simulink model "Hoist_raw"  (R2015b)
settings: Solver=ode23t  StartTime=0.0  StopTime=10  MaxStep=0.2  RelTol=1e-3
undefined symbols (not defined in the file or in its folder): sigbuilder_block
libraries: fl_lib x16, nesl_utility x4
settings Model: Creator=OlgeirMac  LastModifiedBy=OlgeirMac
settings SolverCC: ZeroCrossControl=EnableAll

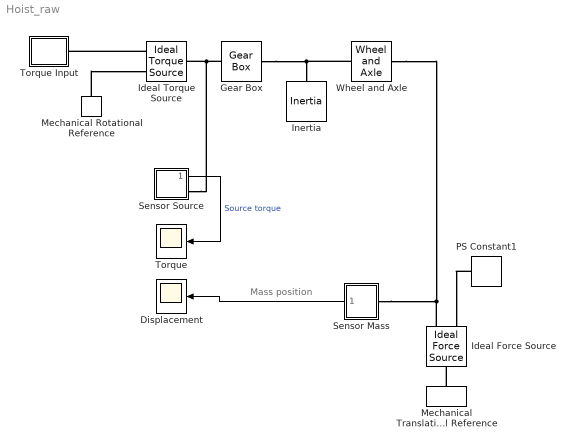
== system Hoist_raw ==
  note: Mass position
  Displacement : Scope
  Gear Box : fl_lib/Mechanical/Mechanisms/Gear Box  ratio=5  t_in_specify=off  t_in_priority=None  t_in=0 N*m  t_out_specify=off  t_out_priority=None  t_out=0 N*m
  Ideal Force Source : fl_lib/Mechanical/Mechanical Sources/Ideal Force Source
  Ideal Torque Source : fl_lib/Mechanical/Mechanical Sources/Ideal Torque Source
  Inertia : fl_lib/Mechanical/Rotational Elements/Inertia  inertia=0.001 kg*m^2  w_specify=off  w_priority=None  w=0 rad/s  t_specify=off  t_priority=None  t=0 N*m
  Mechanical Rotational Reference : fl_lib/Mechanical/Rotational Elements/Mechanical Rotational Reference
  Mechanical Translational Reference : fl_lib/Mechanical/Translational Elements/Mechanical Translational Reference
  PS Constant1 : fl_lib/Physical Signals/Sources/PS Constant  constant=9.8*load
  Sensor Mass : Subsystem
      mask Display: disp('P')
  Sensor Source : Subsystem
      mask Display: disp('P')
  Torque : Scope
  Torque Input : Subsystem
  Wheel and Axle : fl_lib/Mechanical/Mechanisms/Wheel and Axle  R=0.5 m  or=1  orient=1  t_specify=off  t_priority=None  t=0 N*m  f_specify=off  f_priority=None  f=0 N
  wires:
  Sensor Mass/1(Out1) -> Displacement/1
  Sensor Source/1(Out1) -> Torque/1  "Source torque"
  connections:
  Ideal Torque Source/RConn1 -- Torque Input/RConn1
  Gear Box/LConn1 -- Sensor Source/RConn1 -- Ideal Torque Source/LConn1
  Gear Box/RConn1 -- Wheel and Axle/LConn1 -- Inertia/LConn1
  Mechanical Rotational Reference/LConn1 -- Ideal Torque Source/RConn2
  Sensor Mass/LConn1 -- Wheel and Axle/RConn1 -- Ideal Force Source/RConn2
  PS Constant1/RConn1 -- Ideal Force Source/RConn1
  Mechanical Translational Reference/LConn1 -- Ideal Force Source/LConn1

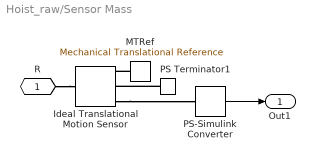
== system Hoist_raw/Sensor Mass ==
  Ideal Translational Motion Sensor : fl_lib/Mechanical/Mechanical Sensors/Ideal Translational Motion Sensor  Tag=Factory Generic  offset=0 m
  MTRef : fl_lib/Mechanical/Translational Elements/Mechanical Translational Reference  Tag=Factory Generic
  PS Terminator1 : fl_lib/Physical Signals/Sinks/PS Terminator
  PS-Simulink Converter : nesl_utility/PS-Simulink Converter  PhysicalDomain=network_engine_domain  SubClassName=ps_output  LeftPortType=input  RightPortType=output  PseudoPeriodic=off  Frequencies=[]  Unit=1  AffineConversion=off
  R : PMIOPort  Port=1  Side=Left
  Out1 : Outport
  wires:
  PS-Simulink Converter/1 -> Out1/1
  connections:
  Ideal Translational Motion Sensor/RConn3 -- PS-Simulink Converter/LConn1
  MTRef/LConn1 -- Ideal Translational Motion Sensor/RConn1
  R/RConn1 -- Ideal Translational Motion Sensor/LConn1
  PS Terminator1/LConn1 -- Ideal Translational Motion Sensor/RConn2

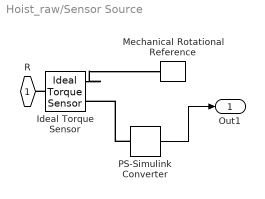
== system Hoist_raw/Sensor Source ==
  Ideal Torque Sensor : fl_lib/Mechanical/Mechanical Sensors/Ideal Torque Sensor
  Mechanical Rotational Reference : fl_lib/Mechanical/Rotational Elements/Mechanical Rotational Reference
  PS-Simulink Converter : nesl_utility/PS-Simulink Converter  PhysicalDomain=network_engine_domain  SubClassName=ps_output  LeftPortType=input  RightPortType=output  PseudoPeriodic=off  Frequencies=[]  Unit=1  AffineConversion=off
  R : PMIOPort  Port=1  Side=Right
  Out1 : Outport
  wires:
  PS-Simulink Converter/1 -> Out1/1
  connections:
  Ideal Torque Sensor/LConn1 -- R/RConn1
  Ideal Torque Sensor/RConn1 -- Mechanical Rotational Reference/LConn1
  PS-Simulink Converter/LConn1 -- Ideal Torque Sensor/RConn2

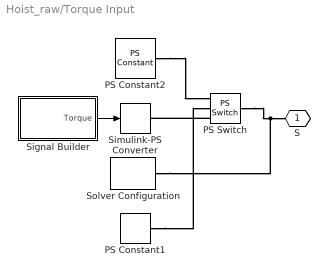
== system Hoist_raw/Torque Input ==
  PS Constant1 : fl_lib/Physical Signals/Sources/PS Constant  constant=2
  PS Constant2 : fl_lib/Physical Signals/Sources/PS Constant  constant=0
  PS Switch : fl_lib/Physical Signals/Nonlinear Operators/PS Switch  Threshold=1
  Signal Builder : Subsystem  Tag=STV Subsys  LoadFcn=sigbuilder_block('load');  StartFcn=sigbuilder_block('start');  StopFcn=sigbuilder_block('stop');  ClipboardFcn=sigbuilder_block('clipboard');  mask(Sigbuilder block){}
      mask help: Sigbuilder GUI
      mask init:
      | if ~strcmp(get_param(bdroot(gcbh),'SimulationStatus'),'stopped') tuvar = sigbuilder_block('maskInit'); end
      settings: CopyFcn=sigbuilder_block('copy');  DeleteFcn=sigbuilder_block('delete');  ModelCloseFcn=sigbuilder_block('modelClose');  PreSaveFcn=sigbuilder_block('preSave');  PauseFcn=sigbuilder_block('pause')  ContinueFcn=sigbuilder_block('continue')  NameChangeFcn=sigbuilder_block('namechange');  OpenFcn=sigbuilder_block('open',[559 266 585 292 ]);  CloseFcn=sigbuilder_block('close');
      mask Display: plot(0,0,100,100,[10,10,40,40,10],[80,20,20,80,80],[40,10],[50,50], [40,27,10],[65,72,56],[40,25,25,10],[28,28,43,43]);
  Simulink-PS Converter : nesl_utility/Simulink-PS Converter  PhysicalDomain=network_engine_domain  SubClassName=ps_input  LeftPortType=input  RightPortType=output  PseudoPeriodic=off  Frequencies=[]  NoiseDistribution=none  NoiseParameters=[]  Unit=1  AffineConversion=off  InputFiltering=off  SimscapeFilterOrder=1  InputFilterTimeConstant=.001  UdotUserProvided=[]
  Solver Configuration : nesl_utility/Solver Configuration  PhysicalDomain=network_engine_domain  SubClassName=solver  LeftPortType=input  RightPortType=generic  Accelerate=off  Tones=[]  Harmonics=[]  SimulateNoise=off  Profile=off  UseLocalSampling=off  EnableSwitchedLinearOptims=on  FrequencyDomain=off  UseCCode=off  RelTol=0.001  AbsTol=1e-06  MinStep=1e-09  ToWorkspace=off  RevertToSquareIcSolve=off  NumHomotopyIterations=100  PhasorMode=off  PhasorModeNumHarmonics=1  DoDC=off  ResidualTolerance=1e-9  UseLocalSolver=off  LocalSolverChoice=NE_BACKWARD_EULER_ADVANCER  LocalSolverSampleTime=.001  DoFixedCost=off  MaxNonlinIter=3  MaxModeIter=2  LinearAlgebra=Sparse  DelaysMemoryBudget=1024  AutomaticFiltering=on  FilteringTimeConstant=0.001
  S : PMIOPort  Port=1  Side=Right
  wires:
  Signal Builder/1(Torque) -> Simulink-PS Converter/1
  connections:
  PS Switch/LConn3 -- Simulink-PS Converter/RConn1
  PS Constant2/RConn1 -- PS Switch/LConn1
  PS Switch/RConn1 -- Solver Configuration/RConn1 -- S/RConn1
  PS Constant1/RConn1 -- PS Switch/LConn2

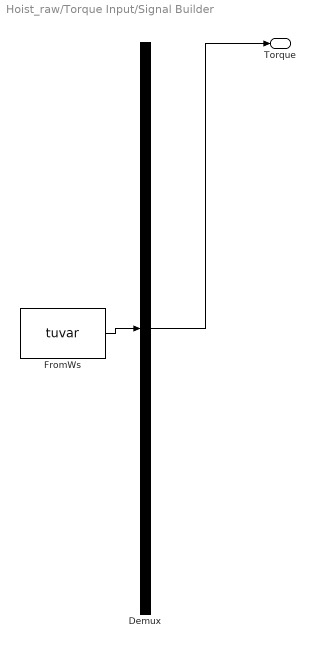
== system Hoist_raw/Torque Input/Signal Builder ==
  Demux : Demux  Tag=STV Demux  Outputs=1
  FromWs : FromWorkspace  Tag=STV FromWs  VariableName=tuvar  SampleTime=0
      SigBuilderData=|
      | common.afterFinalStr = 'Extrapolate'
      | common.sampleTime = 0
      | dataSet.timeRange = [0 40]
      | dataSet.name = 'Group 1'
      | sbobj.Groups.Name = 'Group 1'
      | sbobj.Groups.Signals.Name = 'Torque'
      | sbobj.Groups.Signals.XData = [0 0.1 0.2 0.2 2.1 2.1 2.2 2.2 6.1 6.1 6.3 6.3 11.1 11.3 17 17.2 17.2 24.1 24.1 24.5 24.5 32.1 32.1 32.7 36.85 37.35 40]
      | sbobj.Groups.Signals.YData = [-0.01 -0.01 0.4 0.38 0.38 0.37 -0.02 0.8 0.85 0 0 0.015 0 0.01 0.01 0.02 0.01 0.01 0.4 -0.38 0.01 -0.01 -0.4 0.4 0.4 0 0]
      | sbobj.Groups.TimeRange = [0 40]
  Torque : Outport  Tag=STV Outport
  wires:
  Demux/1 -> Torque/1
  FromWs/1 -> Demux/1
